simulink model "encoder1_ver2"  (R2021b)
settings: Solver=FixedStepAuto  StartTime=0.0  StopTime=inf  RelTol=1e-3  EnableMultiTasking=on
libraries: arduinolib x21, arduinosensorlib x10, fuzblock x4
settings Model: ExtModeTrigDuration=2  Creator=Admin  LastModifiedBy=LENOVO
settings SolverCC: AutoInsertRateTranBlk=on
settings OptimizationCC: EnhancedBackFolding=on  PassReuseOutputArgsAs=Individual arguments  ZeroExternalMemoryAtStartup=off  ZeroInternalMemoryAtStartup=off  MaxStackSize=64  OptimizeBlockOrder=speed  DifferentSizesBufferReuse=on  OptimizationCustomize=off  EfficientTunableParamExpr=on
settings DebuggingCC: ParameterTunabilityLossMsg=error
settings HardwareCC: ProdBitPerInt=16  ProdBitPerPointer=16  ProdBitPerSizeT=16  ProdBitPerPtrDiffT=16  ProdLargestAtomicFloat=None  ProdWordSize=8  ProdHWDeviceType=Atmel->AVR
settings SFSimCC: MATLABDynamicMemAlloc=off
settings RTWCC: Description=Embedded Coder  SystemTargetFile=ert.tlc  HardwareBoard=Arduino Mega 2560  TemplateMakefile=ert_default_tmf  Toolchain=Arduino AVR  BuildConfiguration=Faster Runs
settings CodeAppCC: ForceParamTrailComments=on  IgnoreCustomStorageClasses=off  OperatorAnnotations=on  SimulinkDataObjDesc=on  SFDataObjDesc=on  InsertBlockDesc=on
settings ERTTargetCC: SupportContinuousTime=on  SupportVariableSizeSignals=on  ExtModeTransport=3  ExtModeStaticAlloc=on  ExtModeStaticAllocSize=2048  ExtModeMexFile=ext_xcp  ExtModeIntrfLevel=Level2 - Open

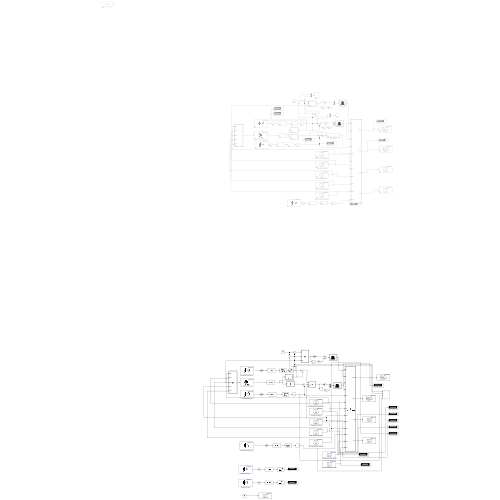
[thumbnail: Simulink's stored preview of the top-level diagram]
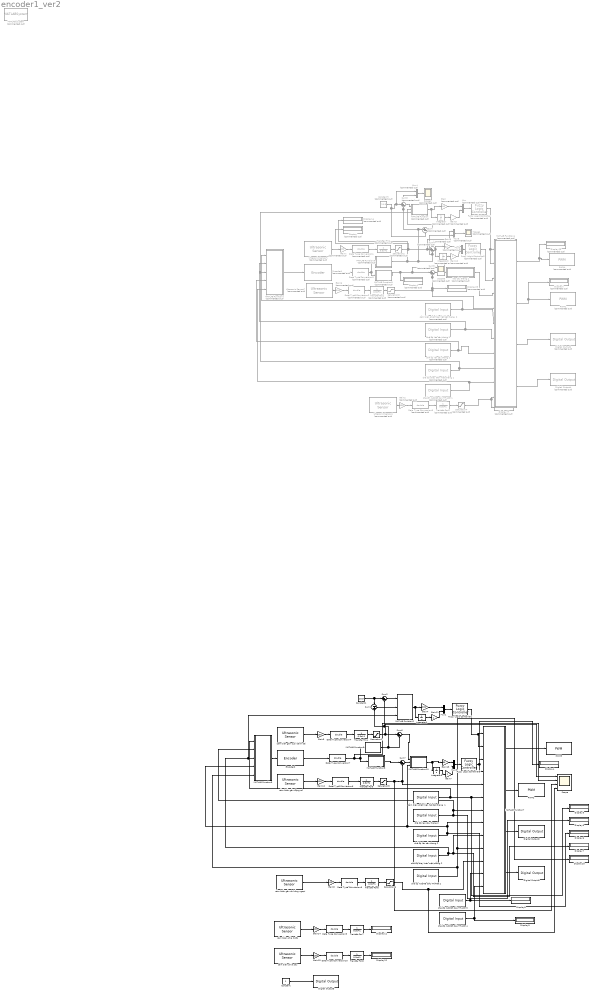
== system encoder1_ver2 ==
  "  chế độ XUỐNG CẦU THANG 1" : arduinolib/Digital Input  Commented=on  pinNumber=36  mode=Default  Direction=input  SampleTime=0.1  blockPlatform=arduino
  "  chế độ XUỐNG CẦU THANG 2" : arduinolib/Digital Input  pinNumber=36  mode=Default  Direction=input  SampleTime=0.1  blockPlatform=arduino
  "  chế độ XUỐNG CẦU THANG 3" : arduinolib/Digital Input  pinNumber=38  mode=Default  Direction=input  SampleTime=0.1  blockPlatform=arduino
  "  chế độ XUỐNG CẦU THANG 4" : arduinolib/Digital Input  pinNumber=40  mode=Default  Direction=input  SampleTime=0.1  blockPlatform=arduino
  "  chế độ chạy trên mặt phẳng 1" : arduinolib/Digital Input  Commented=on  pinNumber=34  mode=Default  Direction=input  SampleTime=0.1  blockPlatform=arduino
  "  chế độ chạy trên mặt phẳng 2" : arduinolib/Digital Input  pinNumber=34  mode=Default  Direction=input  SampleTime=0.1  blockPlatform=arduino
  "  chế độ leo cầu thang 1" : arduinolib/Digital Input  Commented=on  pinNumber=28  mode=Default  Direction=input  SampleTime=0.1  blockPlatform=arduino
  "  chế độ leo cầu thang 2" : arduinolib/Digital Input  pinNumber=28  mode=Default  Direction=input  SampleTime=0.1  blockPlatform=arduino
  "  chế độ lên cầu thang 1" : arduinolib/Digital Input  Commented=on  pinNumber=30  mode=Default  Direction=input  SampleTime=0.1  blockPlatform=arduino
  "  chế độ lên cầu thang 2" : arduinolib/Digital Input  pinNumber=30  mode=Default  Direction=input  SampleTime=0.1  blockPlatform=arduino
  "  cảm biến phát hiện hết bật thang  1" : arduinolib/Digital Input  pinNumber=26  mode=Default  Direction=input  SampleTime=0.1  blockPlatform=arduino
  "  cảm biến phát hiện hết bật thang  2" : arduinolib/Digital Input  Commented=on  pinNumber=26  mode=Default  Direction=input  SampleTime=0.1  blockPlatform=arduino
  Constant : Constant
  Constant1 : Constant  Value=10.5
  Constant2 : Constant  Commented=on  Value=11.5
  Data Type Conversion{1..3,5} (4 alike) : DataTypeConversion  Commented=on  OutDataTypeStr=double
  Data Type Conversion{4,6..10} (6 alike) : DataTypeConversion  OutDataTypeStr=double
  Digital Output1 : arduinolib/Digital Output  Commented=on  pinNumber=22  Direction=output  blockPlatform=arduino
  Digital Output2 : arduinolib/Digital Output  pinNumber=22  Direction=output  blockPlatform=arduino
  Digital Output3 : arduinolib/Digital Output  pinNumber=24  Direction=output  blockPlatform=arduino
  Digital Output4 : arduinolib/Digital Output  Commented=on  pinNumber=24  Direction=output  blockPlatform=arduino
  Digital Output5 : arduinolib/Digital Output  pinNumber=46  Direction=output  blockPlatform=arduino
  Display{,1..2,14,17,23,25} (7 alike) : Display  Commented=on
  Display{3..12} (10 alike) : Display
  Encoder1 : arduinosensorlib/Encoder  Commented=on  InputA=2  InputB=3  Mode=Reset by external signal  SampleTime=0.1
      settings: SourceProductBaseCode=ARDUINO
  Encoder2 : arduinosensorlib/Encoder  InputA=2  InputB=3  Mode=Reset by external signal  SampleTime=0.1
      settings: SourceProductBaseCode=ARDUINO
  Fuzzy Logic Controller : fuzblock/Fuzzy Logic  Controller  Commented=on  FIS='dkm7.fis'  OutputSampleNumber=101  DataType=double  FuzzifiedInputs=off  RuleFiringStrengths=off  RuleOutputs=off  AggregatedOutputs=off  SimulateUsing=Interpreted execution  OutOfRangeInputValueMessage=warning  NoRuleFiredMessage=warning  EmptyOutputFuzzySetMessage=warning
  Fuzzy Logic Controller1 : fuzblock/Fuzzy Logic  Controller  FIS='thich_nghi_9_luat.fis'  OutputSampleNumber=101  DataType=double  FuzzifiedInputs=off  RuleFiringStrengths=off  RuleOutputs=off  AggregatedOutputs=off  SimulateUsing=Interpreted execution  OutOfRangeInputValueMessage=warning  NoRuleFiredMessage=warning  EmptyOutputFuzzySetMessage=warning
  Fuzzy Logic Controller2 : fuzblock/Fuzzy Logic  Controller  Commented=on  FIS='dkm7.fis'  OutputSampleNumber=101  DataType=double  FuzzifiedInputs=off  RuleFiringStrengths=off  RuleOutputs=off  AggregatedOutputs=off  SimulateUsing=Interpreted execution  OutOfRangeInputValueMessage=warning  NoRuleFiredMessage=warning  EmptyOutputFuzzySetMessage=warning
  Fuzzy Logic Controller3 : fuzblock/Fuzzy Logic  Controller  FIS='thich_nghi_9_luat.fis'  OutputSampleNumber=101  DataType=double  FuzzifiedInputs=off  RuleFiringStrengths=off  RuleOutputs=off  AggregatedOutputs=off  SimulateUsing=Interpreted execution  OutOfRangeInputValueMessage=warning  NoRuleFiredMessage=warning  EmptyOutputFuzzySetMessage=warning
  Gain : Gain  Commented=on  Gain=500
  Gain1 : Gain  Commented=on  Gain=100
  Gain10 : Gain  Commented=on
  Gain11 : Gain
  Gain{5,8,12,14..15} (5 alike) : Gain  Gain=100
  Gain13 : Gain  Gain=50
  Gain2 : Gain  Commented=on  Gain=100
  Gain3 : Gain  Commented=on  Gain=0.01
  Gain4 : Gain  Gain=200
  Gain6 : Gain  Commented=on  Gain=100
  Gain7 : Gain
  Gain9 : Gain  Commented=on  Gain=50
  Integrator : Integrator  Commented=on
  Integrator1 : Integrator
  Integrator2 : Integrator  Commented=on
  Integrator3 : Integrator
  MATLAB Function : MATLAB Function  Commented=on  TreatAsAtomicUnit=on
  MATLAB Function1 : MATLAB Function  Commented=on  TreatAsAtomicUnit=on
  MATLAB Function10 : MATLAB Function  TreatAsAtomicUnit=on
  MATLAB Function2 : MATLAB Function  TreatAsAtomicUnit=on
  MATLAB Function3 : MATLAB Function  Commented=on  TreatAsAtomicUnit=on
  MATLAB Function4 : MATLAB Function  Commented=on  TreatAsAtomicUnit=on
  MATLAB Function5 : MATLAB Function  TreatAsAtomicUnit=on
  MATLAB Function6 : MATLAB Function  TreatAsAtomicUnit=on
  MATLAB Function7 : MATLAB Function  TreatAsAtomicUnit=on
  MATLAB Function8 : MATLAB Function  TreatAsAtomicUnit=on
  MATLAB Function9 : MATLAB Function  Commented=on  TreatAsAtomicUnit=on
  MATLAB System : MATLABSystem  Commented=on  System=Encoder_arduino  Encoder=0  PinA=2  PinB=3  SampleTime=0.1
      mask Type: Encoder_arduino
      mask Display:
      | disp('Encoder');
      | port_label('output',1,'y');
  Mux{,2,4..5} (4 alike) : Mux  Commented=on  Inputs=2
  Mux1 : Mux  Inputs=2
  Mux3 : Mux  Inputs=2
  PWM1 : arduinolib/PWM  Commented=on  pinNumber=7  frequencyType=Default  desiredFrequency=490.2  achievableFrequency=490.2
  PWM2 : arduinolib/PWM  pinNumber=7  frequencyType=Default  desiredFrequency=490.2  achievableFrequency=490.2
  PWM3 : arduinolib/PWM  pinNumber=6  frequencyType=Default  desiredFrequency=490.2  achievableFrequency=490.2
  PWM4 : arduinolib/PWM  Commented=on  pinNumber=6  frequencyType=Default  desiredFrequency=490.2  achievableFrequency=490.2
  Saturation1 : Saturate  UpperLimit=25  LowerLimit=-25
  Saturation2 : Saturate  Commented=on  UpperLimit=25  LowerLimit=-25
  Saturation3 : Saturate  Commented=on  UpperLimit=30  LowerLimit=-30
  Saturation4 : Saturate  Commented=on  UpperLimit=150  LowerLimit=-150
  Saturation5 : Saturate  UpperLimit=30  LowerLimit=-30
  Saturation6 : Saturate  UpperLimit=150  LowerLimit=-150
  Scope : Scope  NumInputPorts=4
  Scope1 : Scope  Commented=on
  Scope2 : Scope  Commented=on
  Scope6 : Scope  Commented=on  NumInputPorts=2
  Sum{,3..5} (4 alike) : Sum  Commented=on  Inputs=|+-
  Sum1 : Sum  Inputs=-+
  Sum2 : Sum  Inputs=|+-
  Sum6 : Sum  Inputs=|+-
  Sum7 : Sum  Inputs=|+-
  Transfer Fcn1 : TransferFcn  Commented=on  Denominator=[0.3 1]
  Transfer Fcn2 : TransferFcn  Commented=on  Denominator=[0.3 1]
  Transfer Fcn3 : TransferFcn  Commented=on  Denominator=[0.3 1]
  Transfer Fcn4 : TransferFcn  Denominator=[0.3 1]  ParameterTunability=Optimized
  Transfer Fcn{5..8} (4 alike) : TransferFcn  Denominator=[0.3 1]
  Ultrasonic Sensor1 : arduinosensorlib/Ultrasonic Sensor  Commented=on  NumSignalPins=2  TrigPin=8  EchoPin=9  SignalPin=3  SampleTime_=0.1  blockPlatform=ARDUINO
      settings: SourceProductBaseCode=ARDUINO
  Ultrasonic Sensor2 : arduinosensorlib/Ultrasonic Sensor  Commented=on  NumSignalPins=2  TrigPin=10  EchoPin=11  SignalPin=3  SampleTime_=0.1  blockPlatform=ARDUINO
      settings: SourceProductBaseCode=ARDUINO
  Ultrasonic Sensor4 : arduinosensorlib/Ultrasonic Sensor  Commented=on  NumSignalPins=2  TrigPin=4  EchoPin=5  SignalPin=3  SampleTime_=0.1  blockPlatform=ARDUINO
      settings: SourceProductBaseCode=ARDUINO
  cảm biến gần cb hồng ngoại : arduinosensorlib/Ultrasonic Sensor  NumSignalPins=2  TrigPin=4  EchoPin=5  SignalPin=3  SampleTime_=0.1  blockPlatform=ARDUINO
      settings: SourceProductBaseCode=ARDUINO
  cảm biến gần cuối bánh đai : arduinosensorlib/Ultrasonic Sensor  NumSignalPins=2  TrigPin=8  EchoPin=9  SignalPin=3  SampleTime_=0.1  blockPlatform=ARDUINO
      settings: SourceProductBaseCode=ARDUINO
  cảm biến gần động cơ : arduinosensorlib/Ultrasonic Sensor  NumSignalPins=2  TrigPin=10  EchoPin=11  SignalPin=3  SampleTime_=0.1  blockPlatform=ARDUINO
      settings: SourceProductBaseCode=ARDUINO
  cảm biến phía sau : arduinosensorlib/Ultrasonic Sensor  NumSignalPins=2  TrigPin=48  EchoPin=50  SignalPin=3  SampleTime_=0.1  blockPlatform=ARDUINO
      settings: SourceProductBaseCode=ARDUINO
  cảm biến phía trước : arduinosensorlib/Ultrasonic Sensor  NumSignalPins=2  TrigPin=44  EchoPin=42  SignalPin=3  SampleTime_=0.1  blockPlatform=ARDUINO
      settings: SourceProductBaseCode=ARDUINO
  leo cầu thang 1 : Subsystem  Commented=on
  wires:
  Gain/1 -> Mux/1
  Gain3/1 -> Mux/2
  Mux/1 -> Fuzzy Logic Controller/1
  Integrator/1 -> Gain3/1
  "  chế độ XUỐNG CẦU THANG 1"/1 -> MATLAB Function1/5(data4), MATLAB Function4/10(data3)
  "  chế độ leo cầu thang 1"/1 -> MATLAB Function1/2(data2), MATLAB Function4/7(data)
  Saturation2/1 -> Mux5/1, Sum4/1, Display/1
  Data Type Conversion1/1 -> Transfer Fcn1/1
  MATLAB Function4/1(PWMR) -> Display23/1, PWM4/1
  "  cảm biến phát hiện hết bật thang  2"/1 -> MATLAB Function1/1(data), MATLAB Function4/6(TC)
  Ultrasonic Sensor1/1 -> Gain1/1
  Transfer Fcn1/1 -> Saturation2/1
  "  chế độ lên cầu thang 1"/1 -> MATLAB Function4/8(data2), MATLAB Function1/4(data1)
  MATLAB Function4/4(ENL) -> Digital Output4/1
  MATLAB Function4/3(ENR) -> Digital Output1/1
  "  chế độ chạy trên mặt phẳng 1"/1 -> MATLAB Function/3(data), MATLAB Function1/3(data3), MATLAB Function4/9(data5)
  Gain1/1 -> Data Type Conversion1/1
  MATLAB Function1/1(y) -> Encoder1/1
  MATLAB Function4/2(PWML) -> Display2/1, PWM1/1
  Data Type Conversion2/1 -> Transfer Fcn2/1
  Gain6/1 -> Data Type Conversion2/1
  Ultrasonic Sensor2/1 -> Gain6/1
  Transfer Fcn2/1 -> Saturation3/1
  Encoder1/1 -> Data Type Conversion3/1
  Data Type Conversion3/1 -> MATLAB Function9/1(u), MATLAB Function3/1(u)
  Gain2/1 -> Data Type Conversion5/1
  Data Type Conversion5/1 -> Transfer Fcn3/1
  Ultrasonic Sensor4/1 -> Gain2/1
  Transfer Fcn3/1 -> Saturation4/1
  Saturation4/1 -> Display17/1, MATLAB Function4/11(data4)
  Fuzzy Logic Controller/1 -> MATLAB Function4/2(cm), MATLAB Function4/1(MP)
  Integrator2/1 -> Gain10/1
  Mux2/1 -> Fuzzy Logic Controller2/1
  Gain10/1 -> Mux2/2
  Gain9/1 -> Mux2/1
  Sum4/1 -> Gain9/1, Integrator2/1
  Fuzzy Logic Controller2/1 -> MATLAB Function4/3(u)
  Sum5/1 -> leo cầu thang 1/1(h)
  leo cầu thang 1/1(u) -> MATLAB Function4/4(U1)
  Saturation3/1 -> Scope6/2, Sum5/2, Display25/1, MATLAB Function4/5(data1)
  MATLAB Function3/1(y) -> Mux5/2, Sum4/2, Sum/1, Mux4/2, Sum3/2, Display14/1
  MATLAB Function9/1(y) -> Display1/1, Scope6/1, Sum5/1
  Constant2/1 -> Sum/2, Mux4/1, Sum3/1
  Sum3/1 -> MATLAB Function/1(u)
  Sum/1 -> MATLAB Function/2(u1)
  MATLAB Function/1(y) -> Integrator/1, Gain/1
  Sum2/1 -> MATLAB Function2/1(u)
  MATLAB Function2/1(y) -> Integrator1/1, Gain4/1
  Sum1/1 -> MATLAB Function2/2(u1)
  Constant1/1 -> Sum2/1, Sum1/1
  MATLAB Function8/1(y) -> Sum7/1
  "  chế độ chạy trên mặt phẳng 2"/1 -> MATLAB Function2/3(data), MATLAB Function5/3(data3), Display7/1, MATLAB Function7/9(data5)
  Transfer Fcn5/1 -> Saturation5/1
  MATLAB Function6/1(y) -> Sum6/2, Sum1/2, Sum2/2
  Mux1/1 -> Fuzzy Logic Controller1/1
  MATLAB Function7/1(PWMR) -> PWM3/1
  "  chế độ XUỐNG CẦU THANG 2"/1 -> Display10/1, MATLAB Function7/10(data3), MATLAB Function5/5(data4)
  "  chế độ lên cầu thang 2"/1 -> Display6/1, MATLAB Function7/8(data2), MATLAB Function10/3(data), MATLAB Function5/4(data1)
  Data Type Conversion7/1 -> Scope/2, MATLAB Function8/1(u), MATLAB Function6/1(u)
  cảm biến gần động cơ/1 -> Gain12/1
  Saturation6/1 -> Scope/4, MATLAB Function7/11(data4)
  Gain5/1 -> Data Type Conversion4/1
  cảm biến gần cb hồng ngoại/1 -> Gain8/1
  Saturation5/1 -> Scope/3, Sum7/2, MATLAB Function7/5(data1)
  Integrator3/1 -> Gain7/1
  Fuzzy Logic Controller1/1 -> MATLAB Function7/2(cm), MATLAB Function7/1(MP)
  Data Type Conversion8/1 -> Transfer Fcn6/1
  cảm biến gần cuối bánh đai/1 -> Gain5/1
  MATLAB Function7/4(ENL) -> Digital Output3/1
  "  cảm biến phát hiện hết bật thang  1"/1 -> Display3/1, MATLAB Function7/6(TC), MATLAB Function5/1(data)
  MATLAB Function5/1(y) -> Encoder2/1
  Mux3/1 -> Fuzzy Logic Controller3/1
  Gain8/1 -> Data Type Conversion8/1
  Transfer Fcn6/1 -> Saturation6/1
  MATLAB Function7/2(PWML) -> PWM2/1
  MATLAB Function7/3(ENR) -> Digital Output2/1
  Integrator1/1 -> Gain11/1
  Encoder2/1 -> Data Type Conversion7/1
  Data Type Conversion6/1 -> Transfer Fcn5/1
  Transfer Fcn4/1 -> Saturation1/1
  Saturation1/1 -> Scope/1, Sum6/1
  Data Type Conversion4/1 -> Transfer Fcn4/1
  "  chế độ leo cầu thang 2"/1 -> Display5/1, MATLAB Function5/2(data2), MATLAB Function7/7(data)
  Gain11/1 -> Mux1/2
  Gain4/1 -> Mux1/1
  Gain12/1 -> Data Type Conversion6/1
  Sum6/1 -> MATLAB Function10/1(u)
  Sum7/1 -> MATLAB Function10/2(u1)
  MATLAB Function10/1(y) -> Gain13/1, Integrator3/1
  Mux4/1 -> Scope2/1
  Mux5/1 -> Scope1/1
  "  chế độ XUỐNG CẦU THANG 3"/1 -> MATLAB Function7/12(data6), Display8/1
  "  chế độ XUỐNG CẦU THANG 4"/1 -> Display9/1, MATLAB Function7/13(data7)
  Gain7/1 -> Mux3/2
  Gain13/1 -> Mux3/1
  Fuzzy Logic Controller3/1 -> Display4/1, MATLAB Function7/3(u), MATLAB Function7/4(U1)
  Data Type Conversion9/1 -> Transfer Fcn7/1
  cảm biến phía trước/1 -> Gain14/1
  Transfer Fcn7/1 -> Display11/1
  Gain14/1 -> Data Type Conversion9/1
  Data Type Conversion10/1 -> Transfer Fcn8/1
  cảm biến phía sau/1 -> Gain15/1
  Transfer Fcn8/1 -> Display12/1
  Gain15/1 -> Data Type Conversion10/1
  Constant/1 -> Digital Output5/1

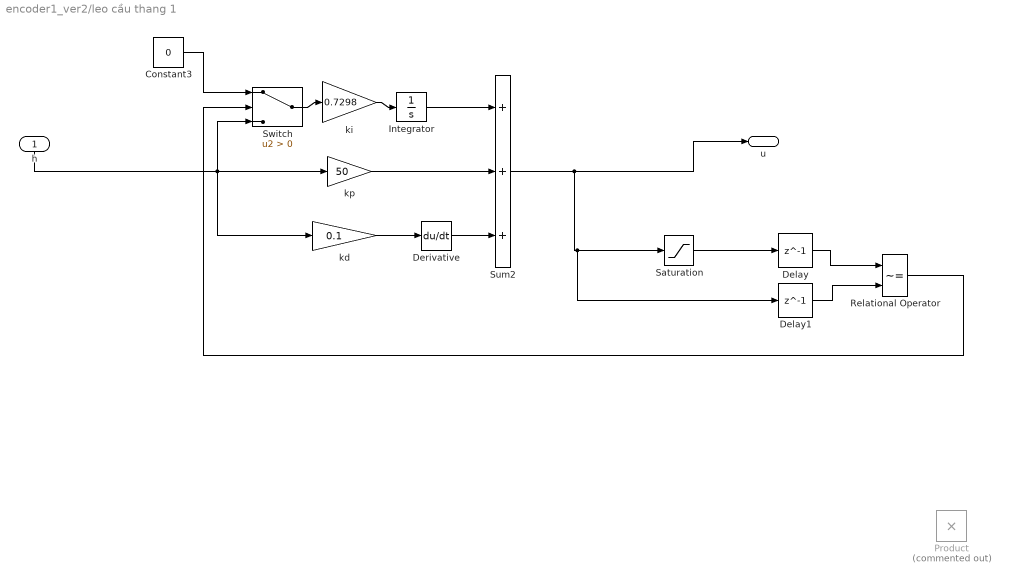
== system encoder1_ver2/leo cầu thang 1 ==
  h : Inport
  Constant3 : Constant  Value=0
  Delay : Delay  DelayLength=1  InitialCondition=0  SampleTime=0.1
  Delay1 : Delay  DelayLength=1  InitialCondition=0  SampleTime=0.1
  Derivative : Derivative
  Integrator : Integrator
  Product : Product  Commented=on
  Relational Operator : RelationalOperator  Operator=~=  OutDataTypeStr=boolean  RndMeth=Simplest
  Saturation : Saturate  UpperLimit=230  LowerLimit=-10
  Sum2 : Sum  Inputs=+++  InputSameDT=on  SaturateOnIntegerOverflow=on  OutDataTypeStr=Inherit: Same as first input
  Switch : Switch  Criteria=u2 > Threshold
  "kd " : Gain  Gain=0.1  ParamDataTypeStr=double  OutDataTypeStr=double
  ki : Gain  Gain=0.7298  SaturateOnIntegerOverflow=on  OutDataTypeStr=Inherit: Same as input  ParamDataTypeStr=Inherit: Same as input
  "kp " : Gain  Gain=50  ParamDataTypeStr=double  OutDataTypeStr=double
  u : Outport
  wires:
  Derivative/1 -> Sum2/3
  "kd "/1 -> Derivative/1
  Integrator/1 -> Sum2/1
  ki/1 -> Integrator/1
  Saturation/1 -> Delay/1
  Relational Operator/1 -> Switch/2
  Delay/1 -> Relational Operator/1
  Delay1/1 -> Relational Operator/2
  Switch/1 -> ki/1
  Constant3/1 -> Switch/1
  "kp "/1 -> Sum2/2
  Sum2/1 -> u/1, Delay1/1, Saturation/1
  h/1 -> Switch/3, "kp "/1, "kd "/1

== matlab function encoder1_ver2/MATLAB Function5 ==
  data: y output; data input; data2 input; data3 input; data1 input; data4 input
function y = fcn(data, data2, data3, data1, data4)
 if data <=0 && data2 >=1 && data1 <=0  % lên 
     y=0;
 elseif data3 >=1 && data2 <=0 && data1>=1  % mặt phẳng 
     y=0;
 elseif data4 <=0 && data3 <=0 && data1 >=1   % xuống 
     y=0;
 else 
     y=1;
 end

== matlab function encoder1_ver2/MATLAB Function6 ==
  data: u input; y output
function y = fcn(u)

y = sqrt(48^2 + 14^2 - 2*48*14*cosd((u/400)*360)) - 24.5;

== matlab function encoder1_ver2/MATLAB Function7 ==
  data: MP input; cm input; u input; U1 input; data1 input; TC input; data input; data2 input; data5 input; data3 input; PWMR output; PWML output; ENR output; ENL output; data4 input; data6 input; data7 input
function [PWMR,PWML,ENR,ENL]=MATLAB_Function4(MP,cm, u,U1,data1, TC,data,data2 ,data5, data3,data4, data6, data7) 
ENR = 1;
ENL = 1;
% chế độ leo cầu thang
  % lên bật cuối cầu thang 
   if data >=1 && TC <=0 && data2 <=0 && data1>=7   % data2 chế độ lên cầu thang, data là chế độ leo cầu thang  
      PWMR = u ;PWML = 0;
   elseif  data1 >=0 && data1 <=6 && data3 >=1 && TC <=0 && data4 >=25 % bật data chế đọ leo cầu thang về vị trí ban đầu 
       PWML = cm; PWMR = 0;
   % lên bật đầu cầu thang 
   elseif data4 >0 && data4 <=25 && data2 <=0 && TC >=1
        PWMR =0 ;PWML=225;
    %chạy trên mặt phẳng 
    elseif data5 >=1    % data1 chế độ chạy trên mặt phẳng
        PWMR = MP;PWML=0; 
  % XUỐNG CẦU THANG 
   elseif data3 <=0 && data <=0
        PWMR = 225; PWML=0;
   elseif data3 <=0 && data >=1 && data1>=0 && data1 <=13
        PWML = U1;PWMR =0;
   elseif data6 <=0
       PWMR =225 ; PWML=0;
   elseif data7<=0
       PWML =225; PWMR =0;
   else
        PWMR =0 ;PWML =0;
   end
end

== matlab function encoder1_ver2/MATLAB Function8 ==
  data: u input; y output
function y = fcn(u)

y = sqrt(48^2 + 14^2 - 2*48*14*cosd((u/400)*360)) - 27;

== matlab function encoder1_ver2/MATLAB Function9 ==
  data: u input; y output
function y = fcn(u)

y = sqrt(48^2 + 14^2 - 2*48*14*cosd((u/400)*360)) - 29;

== matlab function encoder1_ver2/MATLAB Function10 ==
  data: u input; u1 input; y output; data input
function y = fcn(u,u1, data)
 if data <=0 
     y=u;
 else 
     y= u1;
 end

== matlab function encoder1_ver2/MATLAB Function1 ==
  data: y output; data input; data2 input; data3 input; data1 input; data4 input
function y = fcn(data, data2, data3, data1, data4)
 if data <=0 && data2 >=1 && data1 <=0  % lên 
     y=0;
 elseif data3 >=1 && data2 <=0 && data1>=1  % mặt phẳng 
     y=0;
 elseif data4 <=0 && data3 <=0 && data1 >=1   % xuống 
     y=0;
 else 
     y=1;
 end

== matlab function encoder1_ver2/MATLAB Function ==
  data: u input; u1 input; y output; data input
function  y= fcn(u,u1, data)

 if data >=1
     y=u;
 else
     y=u1;
 end

== matlab function encoder1_ver2/MATLAB Function3 ==
  data: u input; y output
function y = fcn(u)

y = sqrt(48^2 + 14^2 - 2*48*14*cosd((u/400)*360)) - 24;

== matlab function encoder1_ver2/MATLAB Function2 ==
  data: u input; u1 input; y output; data input
function  y= fcn(u,u1, data)

 if data >=1
     y=u;
 else
     y=u1;
 end

== matlab function encoder1_ver2/MATLAB Function4 ==
  data: MP input; cm input; u input; U1 input; data1 input; TC input; data input; data2 input; data5 input; data3 input; PWMR output; PWML output; ENR output; ENL output; data4 input
function [PWMR,PWML,ENR,ENL]=MATLAB_Function4(MP,cm, u,U1,data1, TC,data,data2 ,data5, data3,data4) 
ENR = 1;
ENL = 1;
% chế độ leo cầu thang
  % lên bật cuối cầu thang 
   if data >=1 && TC <=0 && data2 <=0&& data1>=7   % data2 chế độ lên cầu thang, data là chế độ leo cầu thang  
      PWMR = u ;PWML = 0;
   elseif  data1 >=0 && data1 <=6 && data3 >=1 && TC <=0 && data4 >=25 % bật data chế đọ leo cầu thang về vị trí ban đầu 
       PWML = cm; PWMR = 0;
   % lên bật đầu cầu thang 
   elseif data4 >0 && data4 <=25 && data2 <=0 && TC >=1
        PWMR =0 ;PWML=225;
    %chạy trên mặt phẳng 
    elseif data5 >=1    % data1 chế độ chạy trên mặt phẳng
        PWMR = MP;PWML=0; 
   % elseif data5 <=0 &&  data2 <=0 && data <=0 && data3 >=1 % sữa 
       % PWMR = 0;PWML =225;
  % XUỐNG CẦU THANG 
   elseif data3 <=0 && data <=0
        PWMR = 225; PWML=0;
   elseif data3 <=0 && data >=1 && data1>=0 && data1 <=9.5
        PWML = U1;PWMR =0;
   else
        PWMR =0 ;PWML =0;
   end
 
  
end
